simulink model "finishi"  (R2016b)
settings: Solver=ode3  StartTime=0.0  StopTime=850.5  FixedStep=0.01  MaxStep=0.01  RelTol=1e-3  EnableMultiTasking=on
PreLoadFcn:
  | m=5;
  | g=9.8;
  | Jxx=0.1539;
  | Jyy=0.1539;
  | Jzz=0.2634;
  | d=0.4;
  | CT=2.757*10^(-5);
  | CM=4.308*10^(-7);
  | CR=727.36;
  | Wb=173.03;
  | Jm=8.61*10^(-5);
  | Tm=0.0435;
  | Cd=0.712
libraries: simulink x10
settings Model: Creator=StarFly  LastModifiedBy=user
settings DataIOCC: LimitDataPoints=on  SaveFormat=Array
settings OptimizationCC: LifeSpan=inf
settings DebuggingCC: SolverPrmCheckMsg=warning  SFUnexpectedBacktrackingDiag=warning  SFNoUnconditionalDefaultTransitionDiag=warning  SFExecutionAtInitializationDiag=none
settings HardwareCC: ProdBitPerPointer=32  ProdBitPerSizeT=32  ProdBitPerPtrDiffT=32  ProdLargestAtomicFloat=None  ProdIntDivRoundTo=Undefined  ProdEndianess=Unspecified  ProdWordSize=32  ProdHWDeviceType=32-bit Generic
settings ModelReferenceCC: PropagateSignalLabelsOutOfModel=off
settings GRTTargetCC: TargetLangStandard=C89/C90 (ANSI)  GeneratePreprocessorConditionals=Disable all
settings ConfigComp: CovMetricSettings=dw  CovHtmlReporting=on  CovSaveCumulativeToWorkspaceVar=on  CovSaveSingleToWorkspaceVar=on  CovExternalEMLEnable=off  CovSFcnEnable=off

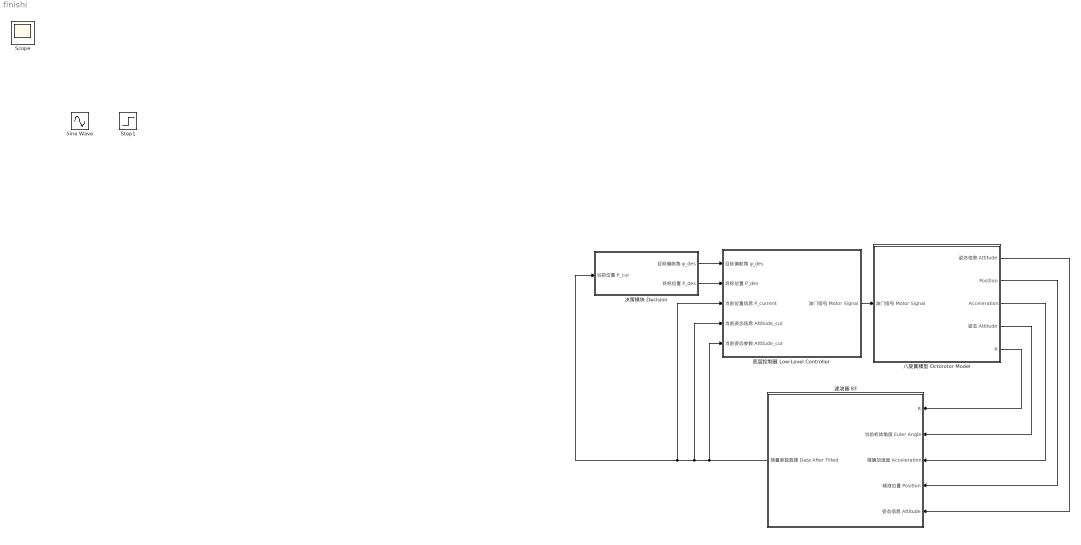
== system finishi ==
  八旋翼模型 Octorotor Model : Subsystem
  决策模块 Decision : Subsystem
  底层控制器 Low-Level Controller : Subsystem
  滤波器 KF : Subsystem
  Scope : Scope
  Sine Wave : Sin  IOType=siggen  SampleTime=0
  Step1 : Step  IOType=siggen  SampleTime=0
  wires:
  滤波器 KF/1(测量参数数据 Data After Filted) -> 底层控制器 Low-Level Controller/4(当前姿态信息 Attitude_cur), 决策模块 Decision/1(当前位置 P_cur), 底层控制器 Low-Level Controller/3(当前位置信息 P_current), 底层控制器 Low-Level Controller/5(当前姿态参数 Attitude_cur)
  八旋翼模型 Octorotor Model/5(R) -> 滤波器 KF/1(R)
  八旋翼模型 Octorotor Model/4(姿态 Attitude) -> 滤波器 KF/2(当前机体角度 Euler Angle)
  八旋翼模型 Octorotor Model/3(Acceleration) -> 滤波器 KF/3(精确加速度 Acceleration)
  八旋翼模型 Octorotor Model/2(Position) -> 滤波器 KF/4(精准位置 Position)
  八旋翼模型 Octorotor Model/1(姿态信息 Attitude) -> 滤波器 KF/5(姿态信息 Attitude)
  决策模块 Decision/1(目标偏航角 ψ_des) -> 底层控制器 Low-Level Controller/1(目标偏航角 ψ_des)
  决策模块 Decision/2(目标位置 P_des) -> 底层控制器 Low-Level Controller/2(目标位置 P_des)
  底层控制器 Low-Level Controller/1(油门信号 Motor Signal) -> 八旋翼模型 Octorotor Model/1(油门信号 Motor Signal)

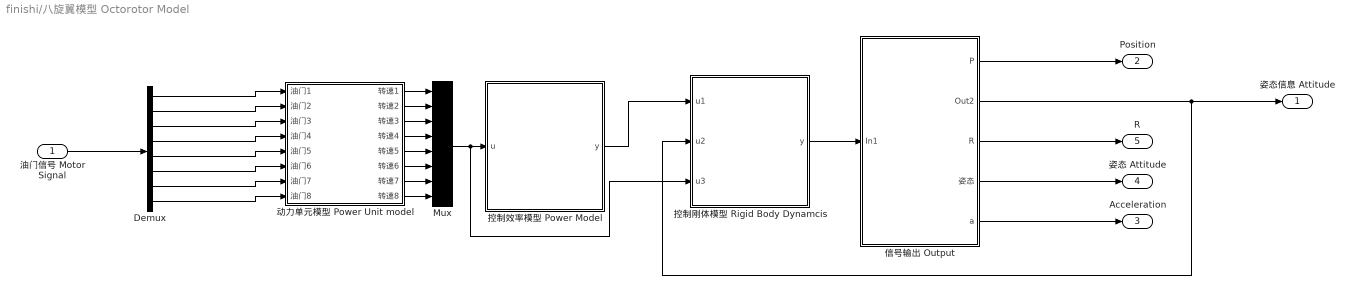
== system finishi/八旋翼模型 Octorotor Model ==
  油门信号 Motor Signal : Inport
  Demux : Demux  Outputs=8
  Mux : Mux  Inputs=8
  信号输出 Output : Subsystem
  动力单元模型 Power Unit model : Subsystem
  控制刚体模型 Rigid Body Dynamcis : MATLAB Function  TreatAsAtomicUnit=on
  控制效率模型 Power Model : MATLAB Function  TreatAsAtomicUnit=on
  姿态信息 Attitude : Outport
  Position : Outport  Port=2
  Acceleration : Outport  Port=3
  姿态 Attitude : Outport  Port=4
  R : Outport  Port=5
  wires:
  动力单元模型 Power Unit model/6(转速6) -> Mux/6
  动力单元模型 Power Unit model/7(转速7) -> Mux/7
  动力单元模型 Power Unit model/8(转速8) -> Mux/8
  动力单元模型 Power Unit model/3(转速3) -> Mux/3
  动力单元模型 Power Unit model/2(转速2) -> Mux/2
  Demux/5 -> 动力单元模型 Power Unit model/5(油门5)
  Mux/1 -> 控制效率模型 Power Model/1(u), 控制刚体模型 Rigid Body Dynamcis/3(u3)
  Demux/3 -> 动力单元模型 Power Unit model/3(油门3)
  Demux/1 -> 动力单元模型 Power Unit model/1(油门1)
  Demux/2 -> 动力单元模型 Power Unit model/2(油门2)
  Demux/6 -> 动力单元模型 Power Unit model/6(油门6)
  动力单元模型 Power Unit model/4(转速4) -> Mux/4
  动力单元模型 Power Unit model/1(转速1) -> Mux/1
  控制效率模型 Power Model/1(y) -> 控制刚体模型 Rigid Body Dynamcis/1(u1)
  Demux/7 -> 动力单元模型 Power Unit model/7(油门7)
  Demux/8 -> 动力单元模型 Power Unit model/8(油门8)
  油门信号 Motor Signal/1 -> Demux/1
  Demux/4 -> 动力单元模型 Power Unit model/4(油门4)
  动力单元模型 Power Unit model/5(转速5) -> Mux/5
  信号输出 Output/2(Out2) -> 控制刚体模型 Rigid Body Dynamcis/2(u2), 姿态信息 Attitude/1
  控制刚体模型 Rigid Body Dynamcis/1(y) -> 信号输出 Output/1(In1)
  信号输出 Output/1(P) -> Position/1
  信号输出 Output/3(R) -> R/1
  信号输出 Output/4(姿态) -> 姿态 Attitude/1
  信号输出 Output/5(a) -> Acceleration/1

== system finishi/决策模块 Decision ==
  当前位置 P_cur : Inport
  Clock : Clock
  决策 Decision : MATLAB Function  TreatAsAtomicUnit=on
  目标psi : Constant  Value=0
  目标偏航角 ψ_des : Outport
  目标位置 P_des : Outport  Port=2
  wires:
  当前位置 P_cur/1 -> 决策 Decision/1(u1)
  Clock/1 -> 决策 Decision/2(u2)
  决策 Decision/1(y) -> 目标位置 P_des/1
  目标psi/1 -> 目标偏航角 ψ_des/1

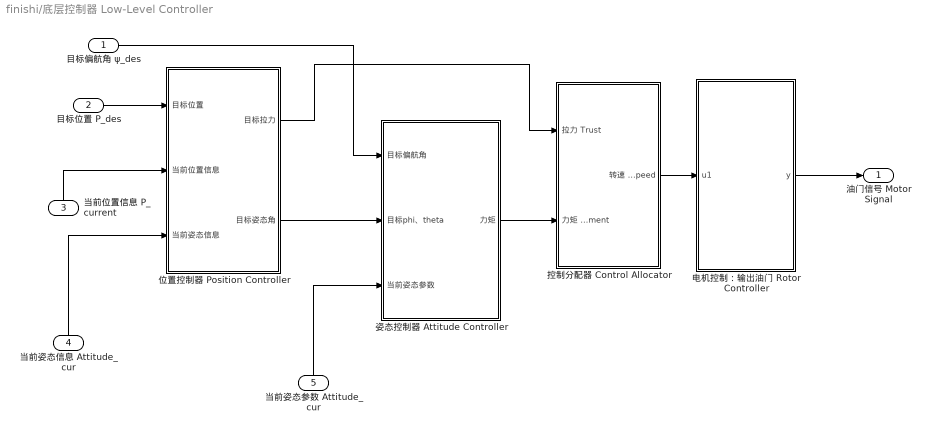
== system finishi/底层控制器 Low-Level Controller ==
  目标偏航角 ψ_des : Inport
  目标位置 P_des : Inport  Port=2
  当前位置信息 P_current : Inport  Port=3
  当前姿态信息 Attitude_cur : Inport  Port=4
  当前姿态参数 Attitude_cur : Inport  Port=5
  位置控制器 Position Controller : Subsystem
  姿态控制器 Attitude Controller : Subsystem
  "控制分配器 Control Allocator " : Subsystem
  电机控制：输出油门 Rotor Controller : MATLAB Function  TreatAsAtomicUnit=on
  油门信号 Motor Signal : Outport
  wires:
  目标偏航角 ψ_des/1 -> 姿态控制器 Attitude Controller/1(目标偏航角)
  目标位置 P_des/1 -> 位置控制器 Position Controller/1(目标位置)
  当前姿态参数 Attitude_cur/1 -> 姿态控制器 Attitude Controller/3(当前姿态参数)
  当前姿态信息 Attitude_cur/1 -> 位置控制器 Position Controller/3(当前姿态信息)
  位置控制器 Position Controller/1(目标拉力) -> "控制分配器 Control Allocator "/1(拉力 Trust)
  位置控制器 Position Controller/2(目标姿态角) -> 姿态控制器 Attitude Controller/2(目标phi、theta)
  当前位置信息 P_current/1 -> 位置控制器 Position Controller/2(当前位置信息)
  姿态控制器 Attitude Controller/1(力矩) -> "控制分配器 Control Allocator "/2("力矩 Moment ")
  电机控制：输出油门 Rotor Controller/1(y) -> 油门信号 Motor Signal/1
  "控制分配器 Control Allocator "/1("转速 Motor speed ") -> 电机控制：输出油门 Rotor Controller/1(u1)

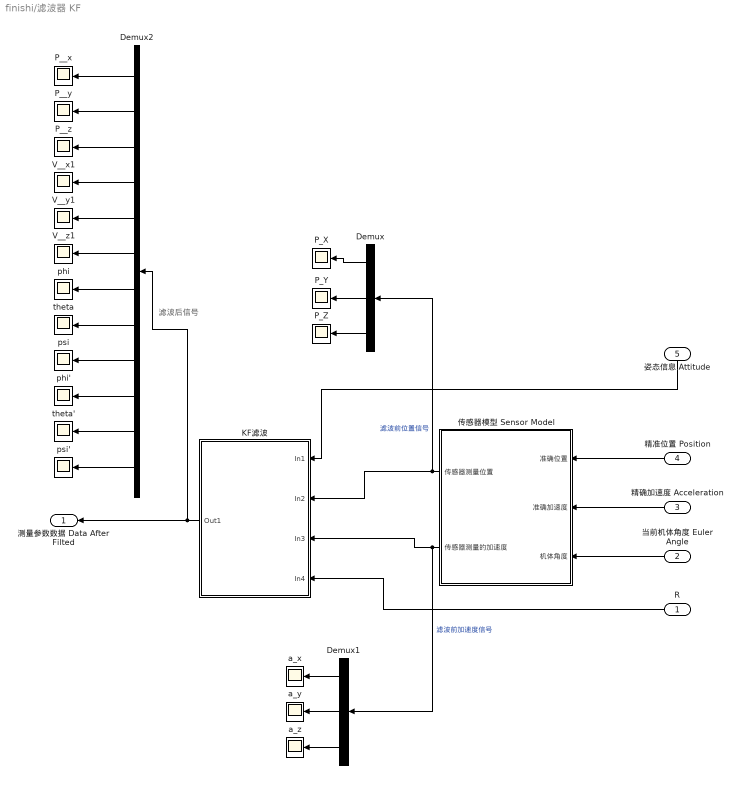
== system finishi/滤波器 KF ==
  note: 滤波后信号
  R : Inport
  当前机体角度 Euler Angle : Inport  Port=2
  精确加速度 Acceleration : Inport  Port=3
  精准位置 Position : Inport  Port=4
  姿态信息 Attitude : Inport  Port=5
  Demux : Demux  Outputs=3
  Demux1 : Demux  Outputs=3
  Demux2 : Demux  Outputs=12
  KF滤波 : Subsystem
  P_X : Scope
  P_Y : Scope
  P_Z : Scope
  P__x : Scope
  P__y : Scope
  P__z : Scope
  V__x1 : Scope
  V__y1 : Scope
  V__z1 : Scope
  a_x : Scope
  a_y : Scope
  a_z : Scope
  phi : Scope
  phi' : Scope
  psi : Scope
  psi' : Scope
  theta : Scope
  theta' : Scope
  传感器模型 Sensor Model : Subsystem
  测量参数数据 Data After Filted : Outport
  wires:
  精准位置 Position/1 -> 传感器模型 Sensor Model/1(准确位置)
  精确加速度 Acceleration/1 -> 传感器模型 Sensor Model/2(准确加速度)
  当前机体角度 Euler Angle/1 -> 传感器模型 Sensor Model/3(机体角度)
  姿态信息 Attitude/1 -> KF滤波/1(In1)
  传感器模型 Sensor Model/1(传感器测量位置) -> Demux/1, KF滤波/2(In2)  "滤波前位置信号"
  R/1 -> KF滤波/4(In4)
  KF滤波/1(Out1) -> Demux2/1, 测量参数数据 Data After Filted/1
  Demux/1 -> P_X/1
  Demux/2 -> P_Y/1
  Demux/3 -> P_Z/1
  传感器模型 Sensor Model/2(传感器测量的加速度) -> Demux1/1, KF滤波/3(In3)  "滤波前加速度信号"
  Demux1/1 -> a_x/1
  Demux1/2 -> a_y/1
  Demux1/3 -> a_z/1
  Demux2/1 -> P__x/1
  Demux2/2 -> P__y/1
  Demux2/3 -> P__z/1
  Demux2/4 -> V__x1/1
  Demux2/5 -> V__y1/1
  Demux2/6 -> V__z1/1
  Demux2/7 -> phi/1
  Demux2/8 -> theta/1
  Demux2/9 -> psi/1
  Demux2/10 -> phi'/1
  Demux2/11 -> theta'/1
  Demux2/12 -> psi'/1

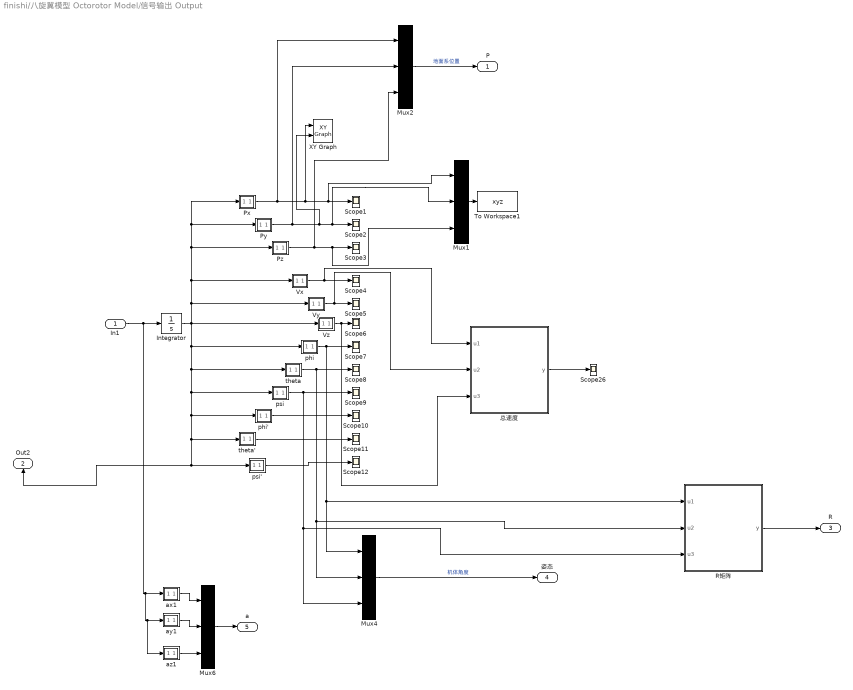
== system finishi/八旋翼模型 Octorotor Model/信号输出 Output ==
  In1 : Inport
  Integrator : Integrator  InitialCondition=[0;0;0;0;0;0;0;0;0;0;0;0]
  Mux{1..2,4,6} (4 alike) : Mux  Inputs=3
  Px : MATLAB Function  TreatAsAtomicUnit=on
  Py : MATLAB Function  TreatAsAtomicUnit=on
  Pz : MATLAB Function  TreatAsAtomicUnit=on
  R矩阵 : MATLAB Function  TreatAsAtomicUnit=on
  Scope{1..12,26} (13 alike) : Scope
  To Workspace1 : ToWorkspace  VariableName=xyz  SampleTime=-1
  Vx : MATLAB Function  TreatAsAtomicUnit=on
  Vy : MATLAB Function  TreatAsAtomicUnit=on
  Vz : MATLAB Function  TreatAsAtomicUnit=on
  XY Graph : simulink/Sinks/XY Graph  xmin=-1  xmax=50  ymin=-1  ymax=120  st=-1
  ax1 : MATLAB Function  TreatAsAtomicUnit=on
  ay1 : MATLAB Function  TreatAsAtomicUnit=on
  az1 : MATLAB Function  TreatAsAtomicUnit=on
  phi : MATLAB Function  TreatAsAtomicUnit=on
  phi' : MATLAB Function  TreatAsAtomicUnit=on
  psi : MATLAB Function  TreatAsAtomicUnit=on
  psi' : MATLAB Function  TreatAsAtomicUnit=on
  theta : MATLAB Function  TreatAsAtomicUnit=on
  theta' : MATLAB Function  TreatAsAtomicUnit=on
  "总速度 " : MATLAB Function  TreatAsAtomicUnit=on
  P : Outport
  Out2 : Outport  Port=2
  R : Outport  Port=3
  姿态 : Outport  Port=4
  a : Outport  Port=5
  wires:
  Vx/1(y) -> "总速度 "/1(u1), Scope4/1
  theta'/1(y) -> Scope11/1
  In1/1 -> az1/1(u), ay1/1(u), ax1/1(u), Integrator/1
  Py/1(y) -> Mux2/2, XY Graph/2, Mux1/2, Scope2/1
  Vy/1(y) -> Scope5/1, "总速度 "/2(u2)
  phi'/1(y) -> Scope10/1
  Vz/1(y) -> "总速度 "/3(u3), Scope6/1
  phi/1(y) -> R矩阵/1(u1), Mux4/1, Scope7/1
  psi/1(y) -> R矩阵/3(u3), Mux4/3, Scope9/1
  Pz/1(y) -> Mux2/3, Mux1/3, Scope3/1
  theta/1(y) -> R矩阵/2(u2), Mux4/2, Scope8/1
  Px/1(y) -> Mux2/1, XY Graph/1, Mux1/1, Scope1/1
  psi'/1(y) -> Scope12/1
  "总速度 "/1(y) -> Scope26/1
  Integrator/1 -> Out2/1, psi'/1(u), theta'/1(u), phi'/1(u), psi/1(u), theta/1(u), phi/1(u), Vz/1(u), Vx/1(u), Px/1(u), Py/1(u), Pz/1(u), Vy/1(u)
  Mux2/1 -> P/1  "地面系位置"
  Mux6/1 -> a/1
  R矩阵/1(y) -> R/1
  Mux4/1 -> 姿态/1  "机体角度"
  ay1/1(y) -> Mux6/2
  az1/1(y) -> Mux6/3
  Mux1/1 -> To Workspace1/1
  ax1/1(y) -> Mux6/1

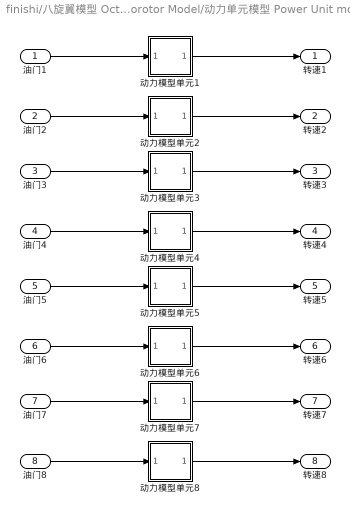
== system finishi/八旋翼模型 Octorotor Model/动力单元模型 Power Unit model ==
  油门1 : Inport
  油门2 : Inport  Port=2
  油门3 : Inport  Port=3
  油门4 : Inport  Port=4
  油门5 : Inport  Port=5
  油门6 : Inport  Port=6
  油门7 : Inport  Port=7
  油门8 : Inport  Port=8
  动力模型单元1 : Subsystem
  动力模型单元2 : Subsystem
  动力模型单元3 : Subsystem
  动力模型单元4 : Subsystem
  动力模型单元5 : Subsystem
  动力模型单元6 : Subsystem
  动力模型单元7 : Subsystem
  动力模型单元8 : Subsystem
  转速1 : Outport
  转速2 : Outport  Port=2
  转速3 : Outport  Port=3
  转速4 : Outport  Port=4
  转速5 : Outport  Port=5
  转速6 : Outport  Port=6
  转速7 : Outport  Port=7
  转速8 : Outport  Port=8
  wires:
  油门1/1 -> 动力模型单元1/1(In1)
  动力模型单元1/1(Out1) -> 转速1/1
  油门2/1 -> 动力模型单元2/1(In1)
  动力模型单元2/1(Out1) -> 转速2/1
  油门3/1 -> 动力模型单元3/1(In1)
  动力模型单元3/1(Out1) -> 转速3/1
  油门4/1 -> 动力模型单元4/1(In1)
  动力模型单元4/1(Out1) -> 转速4/1
  油门5/1 -> 动力模型单元5/1(In1)
  动力模型单元5/1(Out1) -> 转速5/1
  油门6/1 -> 动力模型单元6/1(In1)
  动力模型单元6/1(Out1) -> 转速6/1
  油门7/1 -> 动力模型单元7/1(In1)
  动力模型单元7/1(Out1) -> 转速7/1
  油门8/1 -> 动力模型单元8/1(In1)
  动力模型单元8/1(Out1) -> 转速8/1

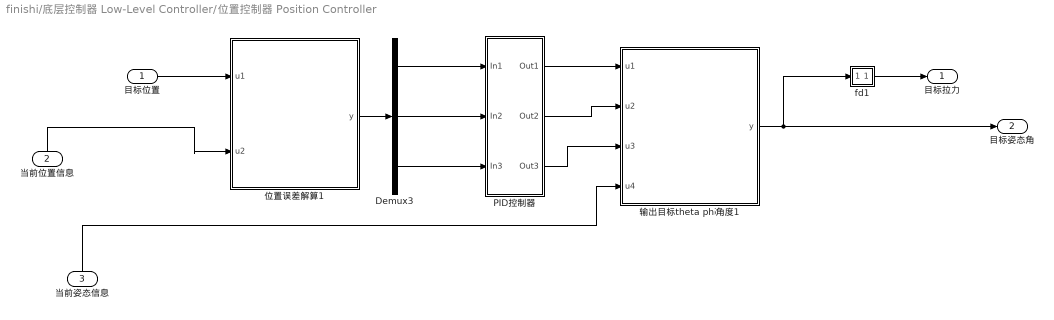
== system finishi/底层控制器 Low-Level Controller/位置控制器 Position Controller ==
  目标位置 : Inport
  当前位置信息 : Inport  Port=2
  当前姿态信息 : Inport  Port=3
  Demux3 : Demux  Outputs=3
  PID控制器 : Subsystem
  fd1 : MATLAB Function  TreatAsAtomicUnit=on
  位置误差解算1 : MATLAB Function  TreatAsAtomicUnit=on
  输出目标theta phi角度1 : MATLAB Function  TreatAsAtomicUnit=on
  目标拉力 : Outport
  目标姿态角 : Outport  Port=2
  wires:
  目标位置/1 -> 位置误差解算1/1(u1)
  fd1/1(y) -> 目标拉力/1
  位置误差解算1/1(y) -> Demux3/1
  输出目标theta phi角度1/1(y) -> fd1/1(u), 目标姿态角/1
  当前位置信息/1 -> 位置误差解算1/2(u2)
  当前姿态信息/1 -> 输出目标theta phi角度1/4(u4)
  Demux3/1 -> PID控制器/1(In1)
  Demux3/2 -> PID控制器/2(In2)
  Demux3/3 -> PID控制器/3(In3)
  PID控制器/1(Out1) -> 输出目标theta phi角度1/1(u1)
  PID控制器/2(Out2) -> 输出目标theta phi角度1/2(u2)
  PID控制器/3(Out3) -> 输出目标theta phi角度1/3(u3)

== system finishi/底层控制器 Low-Level Controller/姿态控制器 Attitude Controller ==
  目标偏航角 : Inport
  目标phi、theta : Inport  Port=2
  当前姿态参数 : Inport  Port=3
  PID控制器 : Subsystem
  姿态误差解算1 : MATLAB Function  TreatAsAtomicUnit=on
  输出目标力矩1 : MATLAB Function  TreatAsAtomicUnit=on
  力矩 : Outport
  wires:
  目标偏航角/1 -> 姿态误差解算1/2(u2)
  当前姿态参数/1 -> 姿态误差解算1/3(u3)
  目标phi、theta/1 -> 姿态误差解算1/1(u1)
  输出目标力矩1/1(y) -> 力矩/1
  姿态误差解算1/1(y) -> PID控制器/1(In1)
  PID控制器/1(Out1) -> 输出目标力矩1/1(u1)
  PID控制器/2(Out2) -> 输出目标力矩1/2(u2)
  PID控制器/3(Out3) -> 输出目标力矩1/3(u3)

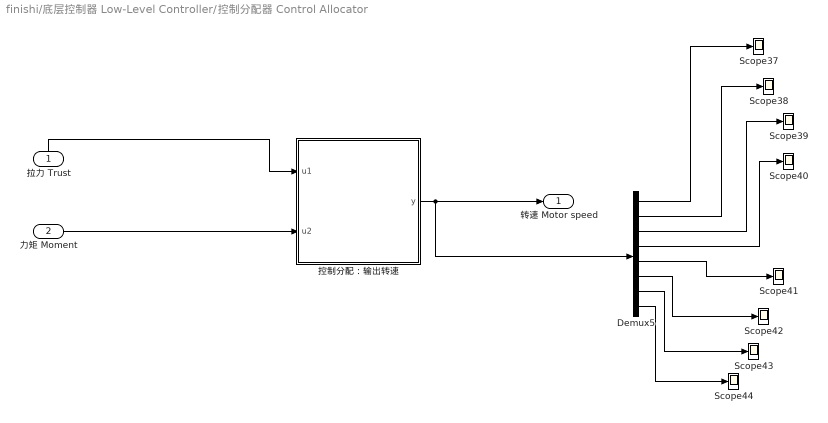
== system finishi/底层控制器 Low-Level Controller/控制分配器 Control Allocator  ==
  拉力 Trust : Inport
  "力矩 Moment " : Inport  Port=2
  Demux5 : Demux  Outputs=8
  Scope{37..44} (8 alike) : Scope
  控制分配：输出转速 : MATLAB Function  TreatAsAtomicUnit=on
  "转速 Motor speed " : Outport
  wires:
  控制分配：输出转速/1(y) -> "转速 Motor speed "/1, Demux5/1
  "力矩 Moment "/1 -> 控制分配：输出转速/2(u2)
  Demux5/1 -> Scope37/1
  Demux5/3 -> Scope39/1
  Demux5/5 -> Scope41/1
  Demux5/8 -> Scope44/1
  Demux5/2 -> Scope38/1
  Demux5/4 -> Scope40/1
  Demux5/7 -> Scope43/1
  Demux5/6 -> Scope42/1
  拉力 Trust/1 -> 控制分配：输出转速/1(u1)

== system finishi/滤波器 KF/KF滤波 ==
  In1 : Inport
  In2 : Inport  Port=2
  In3 : Inport  Port=3
  In4 : Inport  Port=4
  KF : Subsystem
  位置、速度、姿态信息整合 : Subsystem
  Out1 : Outport
  wires:
  KF/1(滤波后位置) -> 位置、速度、姿态信息整合/2(In2)
  In4/1 -> KF/3(R矩阵)
  In3/1 -> KF/2(传感器加速度)
  In2/1 -> KF/1(传感器位置)
  位置、速度、姿态信息整合/1(Out1) -> Out1/1
  KF/2(滤波后速度) -> 位置、速度、姿态信息整合/3(In3)
  In1/1 -> 位置、速度、姿态信息整合/1(In1)

== system finishi/滤波器 KF/传感器模型 Sensor Model ==
  准确位置 : Inport
  准确加速度 : Inport  Port=2
  机体角度 : Inport  Port=3
  GPS模型 : Subsystem
  加速度计模型 : Subsystem
  传感器测量位置 : Outport
  传感器测量的加速度 : Outport  Port=2
  wires:
  准确加速度/1 -> 加速度计模型/1(准确加速度)
  机体角度/1 -> 加速度计模型/2(机体角度)
  加速度计模型/1(传感器测量的加速度) -> 传感器测量的加速度/1
  准确位置/1 -> GPS模型/1(In1)
  GPS模型/1(Out1) -> 传感器测量位置/1

== system finishi/八旋翼模型 Octorotor Model/动力单元模型 Power Unit model/动力模型单元1 ==
  In1 : Inport
  CR : Constant  Value=CR
  Product : Product
  Wb : Constant  Value=Wb
  Wss : Sum
  动态响应 : TransferFcn  Denominator=[Tm 1]
  Out1 : Outport
  wires:
  In1/1 -> Product/2
  Wss/1 -> 动态响应/1
  动态响应/1 -> Out1/1
  Wb/1 -> Wss/1
  CR/1 -> Product/1
  Product/1 -> Wss/2

== system finishi/八旋翼模型 Octorotor Model/动力单元模型 Power Unit model/动力模型单元2 ==
  In1 : Inport
  CR : Constant  Value=CR
  Product : Product
  Wb : Constant  Value=Wb
  Wss : Sum
  动态响应 : TransferFcn  Denominator=[Tm 1]
  Out1 : Outport
  wires:
  Product/1 -> Wss/2
  CR/1 -> Product/1
  Wb/1 -> Wss/1
  动态响应/1 -> Out1/1
  Wss/1 -> 动态响应/1
  In1/1 -> Product/2

== system finishi/八旋翼模型 Octorotor Model/动力单元模型 Power Unit model/动力模型单元3 ==
  In1 : Inport
  CR : Constant  Value=CR
  Product : Product
  Wb : Constant  Value=Wb
  Wss : Sum
  动态响应 : TransferFcn  Denominator=[Tm 1]
  Out1 : Outport
  wires:
  In1/1 -> Product/2
  Wss/1 -> 动态响应/1
  动态响应/1 -> Out1/1
  Wb/1 -> Wss/1
  CR/1 -> Product/1
  Product/1 -> Wss/2

== system finishi/八旋翼模型 Octorotor Model/动力单元模型 Power Unit model/动力模型单元4 ==
  In1 : Inport
  CR : Constant  Value=CR
  Product : Product
  Wb : Constant  Value=Wb
  Wss : Sum
  动态响应 : TransferFcn  Denominator=[Tm 1]
  Out1 : Outport
  wires:
  Product/1 -> Wss/2
  CR/1 -> Product/1
  Wb/1 -> Wss/1
  动态响应/1 -> Out1/1
  Wss/1 -> 动态响应/1
  In1/1 -> Product/2

== system finishi/八旋翼模型 Octorotor Model/动力单元模型 Power Unit model/动力模型单元5 ==
  In1 : Inport
  CR : Constant  Value=CR
  Product : Product
  Wb : Constant  Value=Wb
  Wss : Sum
  动态响应 : TransferFcn  Denominator=[Tm 1]
  Out1 : Outport
  wires:
  In1/1 -> Product/2
  Wss/1 -> 动态响应/1
  动态响应/1 -> Out1/1
  Wb/1 -> Wss/1
  CR/1 -> Product/1
  Product/1 -> Wss/2

== system finishi/八旋翼模型 Octorotor Model/动力单元模型 Power Unit model/动力模型单元6 ==
  In1 : Inport
  CR : Constant  Value=CR
  Product : Product
  Wb : Constant  Value=Wb
  Wss : Sum
  动态响应 : TransferFcn  Denominator=[Tm 1]
  Out1 : Outport
  wires:
  Product/1 -> Wss/2
  CR/1 -> Product/1
  Wb/1 -> Wss/1
  动态响应/1 -> Out1/1
  Wss/1 -> 动态响应/1
  In1/1 -> Product/2

== system finishi/八旋翼模型 Octorotor Model/动力单元模型 Power Unit model/动力模型单元7 ==
  In1 : Inport
  CR : Constant  Value=CR
  Product : Product
  Wb : Constant  Value=Wb
  Wss : Sum
  动态响应 : TransferFcn  Denominator=[Tm 1]
  Out1 : Outport
  wires:
  In1/1 -> Product/2
  Wss/1 -> 动态响应/1
  动态响应/1 -> Out1/1
  Wb/1 -> Wss/1
  CR/1 -> Product/1
  Product/1 -> Wss/2

== system finishi/八旋翼模型 Octorotor Model/动力单元模型 Power Unit model/动力模型单元8 ==
  In1 : Inport
  CR : Constant  Value=CR
  Product : Product
  Wb : Constant  Value=Wb
  Wss : Sum
  动态响应 : TransferFcn  Denominator=[Tm 1]
  Out1 : Outport
  wires:
  Product/1 -> Wss/2
  CR/1 -> Product/1
  Wb/1 -> Wss/1
  动态响应/1 -> Out1/1
  Wss/1 -> 动态响应/1
  In1/1 -> Product/2

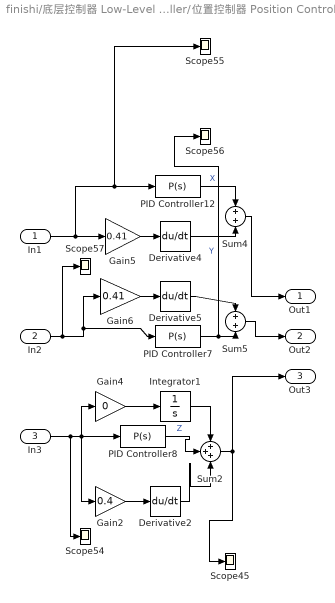
== system finishi/底层控制器 Low-Level Controller/位置控制器 Position Controller/PID控制器 ==
  In1 : Inport
  In2 : Inport  Port=2
  In3 : Inport  Port=3
  Derivative2 : Derivative
  Derivative4 : Derivative  CoefficientInTFapproximation=4.8
  Derivative5 : Derivative
  Gain2 : Gain  Gain=0.4
  Gain4 : Gain  Gain=0
  Gain5 : Gain  Gain=0.41
  Gain6 : Gain  Gain=0.41
  Integrator1 : Integrator
  PID Controller12 : simulink/Continuous/PID Controller  Controller=P  TimeDomain=Continuous-time  SampleTime=-1  IntegratorMethod=Forward Euler  FilterMethod=Forward Euler  Form=Parallel  UseFilter=on  ControllerParametersSource=internal  P=8  I=0  D=1  N=100  InitialConditionSource=internal  InitialConditionForIntegrator=0  InitialConditionForFilter=0  ExternalReset=none  LimitOutput=off  UpperSaturationLimit=inf  LowerSaturationLimit=-inf  LinearizeAsGain=on  AntiWindupMode=none  Kb=1  TrackingMode=off  Kt=1  PParamMin=[]  PParamMax=[]  IParamMin=[]  IParamMax=[]  DParamMin=[]  DParamMax=[]  NParamMin=[]  NParamMax=[]  KbParamMin=[]  KbParamMax=[]  KtParamMin=[]  KtParamMax=[]  POutMin=[]  POutMax=[]  IOutMin=[]  IOutMax=[]  DOutMin=[]  DOutMax=[]  NOutMin=[]  NOutMax=[]  KbOutMin=[]  KbOutMax=[]  KtOutMin=[]  KtOutMax=[]  IntegratorOutMin=[]  IntegratorOutMax=[]  FilterOutMin=[]  FilterOutMax=[]  SumOutMin=[]  SumOutMax=[]  SumI1OutMin=[]  SumI1OutMax=[]  SumI2OutMin=[]  SumI2OutMax=[]  SumI3OutMin=[]  SumI3OutMax=[]  SumDOutMin=[]  SumDOutMax=[]  SaturationOutMin=[]  SaturationOutMax=[]  IntegratorContinuousStateAttributes=''  IntegratorStateMustResolveToSignalObject=off  IntegratorRTWStateStorageClass=Auto  FilterContinuousStateAttributes=''  FilterStateMustResolveToSignalObject=off  FilterRTWStateStorageClass=Auto  DifferentiatorICPrevScaledInput=0  DifferentiatorOutMin=[]  DifferentiatorOutMax=[]
  PID Controller7 : simulink/Continuous/PID Controller  Controller=P  TimeDomain=Continuous-time  SampleTime=-1  IntegratorMethod=Forward Euler  FilterMethod=Forward Euler  Form=Parallel  UseFilter=on  ControllerParametersSource=internal  P=8  I=0  D=1  N=100  InitialConditionSource=internal  InitialConditionForIntegrator=0  InitialConditionForFilter=0  ExternalReset=none  LimitOutput=off  UpperSaturationLimit=inf  LowerSaturationLimit=-inf  LinearizeAsGain=on  AntiWindupMode=none  Kb=1  TrackingMode=off  Kt=1  PParamMin=[]  PParamMax=[]  IParamMin=[]  IParamMax=[]  DParamMin=[]  DParamMax=[]  NParamMin=[]  NParamMax=[]  KbParamMin=[]  KbParamMax=[]  KtParamMin=[]  KtParamMax=[]  POutMin=[]  POutMax=[]  IOutMin=[]  IOutMax=[]  DOutMin=[]  DOutMax=[]  NOutMin=[]  NOutMax=[]  KbOutMin=[]  KbOutMax=[]  KtOutMin=[]  KtOutMax=[]  IntegratorOutMin=[]  IntegratorOutMax=[]  FilterOutMin=[]  FilterOutMax=[]  SumOutMin=[]  SumOutMax=[]  SumI1OutMin=[]  SumI1OutMax=[]  SumI2OutMin=[]  SumI2OutMax=[]  SumI3OutMin=[]  SumI3OutMax=[]  SumDOutMin=[]  SumDOutMax=[]  SaturationOutMin=[]  SaturationOutMax=[]  IntegratorContinuousStateAttributes=''  IntegratorStateMustResolveToSignalObject=off  IntegratorRTWStateStorageClass=Auto  FilterContinuousStateAttributes=''  FilterStateMustResolveToSignalObject=off  FilterRTWStateStorageClass=Auto  DifferentiatorICPrevScaledInput=0  DifferentiatorOutMin=[]  DifferentiatorOutMax=[]
  PID Controller8 : simulink/Continuous/PID Controller  Controller=P  TimeDomain=Continuous-time  SampleTime=-1  IntegratorMethod=Forward Euler  FilterMethod=Forward Euler  Form=Parallel  UseFilter=on  ControllerParametersSource=internal  P=20  I=0  D=1  N=100  InitialConditionSource=internal  InitialConditionForIntegrator=0  InitialConditionForFilter=0  ExternalReset=none  LimitOutput=off  UpperSaturationLimit=inf  LowerSaturationLimit=-inf  LinearizeAsGain=on  AntiWindupMode=none  Kb=1  TrackingMode=off  Kt=1  PParamMin=[]  PParamMax=[]  IParamMin=[]  IParamMax=[]  DParamMin=[]  DParamMax=[]  NParamMin=[]  NParamMax=[]  KbParamMin=[]  KbParamMax=[]  KtParamMin=[]  KtParamMax=[]  POutMin=[]  POutMax=[]  IOutMin=[]  IOutMax=[]  DOutMin=[]  DOutMax=[]  NOutMin=[]  NOutMax=[]  KbOutMin=[]  KbOutMax=[]  KtOutMin=[]  KtOutMax=[]  IntegratorOutMin=[]  IntegratorOutMax=[]  FilterOutMin=[]  FilterOutMax=[]  SumOutMin=[]  SumOutMax=[]  SumI1OutMin=[]  SumI1OutMax=[]  SumI2OutMin=[]  SumI2OutMax=[]  SumI3OutMin=[]  SumI3OutMax=[]  SumDOutMin=[]  SumDOutMax=[]  SaturationOutMin=[]  SaturationOutMax=[]  IntegratorContinuousStateAttributes=''  IntegratorStateMustResolveToSignalObject=off  IntegratorRTWStateStorageClass=Auto  FilterContinuousStateAttributes=''  FilterStateMustResolveToSignalObject=off  FilterRTWStateStorageClass=Auto  DifferentiatorICPrevScaledInput=0  DifferentiatorOutMin=[]  DifferentiatorOutMax=[]
  Scope{45,54..57} (5 alike) : Scope
  Sum2 : Sum  Inputs=+++
  Sum4 : Sum
  Sum5 : Sum
  Out1 : Outport
  Out2 : Outport  Port=2
  Out3 : Outport  Port=3
  wires:
  PID Controller7/1 -> Sum5/2, Scope56/1  "Y"
  In1/1 -> Gain5/1, Scope55/1, PID Controller12/1
  PID Controller8/1 -> Sum2/2  "Z"
  In3/1 -> Scope54/1, Gain4/1, Gain2/1, PID Controller8/1
  PID Controller12/1 -> Sum4/1  "X"
  In2/1 -> Gain6/1, PID Controller7/1, Scope57/1
  Derivative2/1 -> Sum2/3
  Sum2/1 -> Out3/1, Scope45/1
  Gain2/1 -> Derivative2/1
  Derivative5/1 -> Sum5/1
  Gain5/1 -> Derivative4/1
  Gain4/1 -> Integrator1/1
  Gain6/1 -> Derivative5/1
  Sum5/1 -> Out2/1
  Sum4/1 -> Out1/1
  Integrator1/1 -> Sum2/1
  Derivative4/1 -> Sum4/2

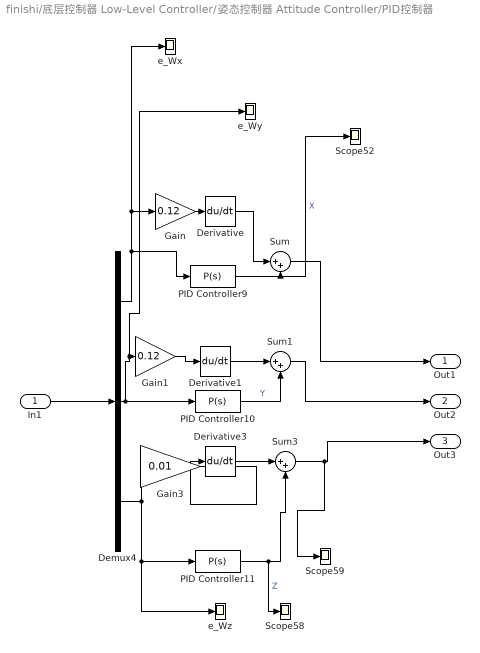
== system finishi/底层控制器 Low-Level Controller/姿态控制器 Attitude Controller/PID控制器 ==
  In1 : Inport
  Demux4 : Demux  Outputs=3
  Derivative : Derivative
  Derivative1 : Derivative
  Derivative3 : Derivative
  Gain : Gain  Gain=0.12
  Gain1 : Gain  Gain=0.12
  Gain3 : Gain  Gain=0.01
  PID Controller10 : simulink/Continuous/PID Controller  Controller=P  TimeDomain=Continuous-time  SampleTime=-1  IntegratorMethod=Forward Euler  FilterMethod=Forward Euler  Form=Parallel  UseFilter=on  ControllerParametersSource=internal  P=8  I=0  D=1  N=100  InitialConditionSource=internal  InitialConditionForIntegrator=0  InitialConditionForFilter=0  ExternalReset=none  LimitOutput=off  UpperSaturationLimit=inf  LowerSaturationLimit=-inf  LinearizeAsGain=on  AntiWindupMode=none  Kb=1  TrackingMode=off  Kt=1  PParamMin=[]  PParamMax=[]  IParamMin=[]  IParamMax=[]  DParamMin=[]  DParamMax=[]  NParamMin=[]  NParamMax=[]  KbParamMin=[]  KbParamMax=[]  KtParamMin=[]  KtParamMax=[]  POutMin=[]  POutMax=[]  IOutMin=[]  IOutMax=[]  DOutMin=[]  DOutMax=[]  NOutMin=[]  NOutMax=[]  KbOutMin=[]  KbOutMax=[]  KtOutMin=[]  KtOutMax=[]  IntegratorOutMin=[]  IntegratorOutMax=[]  FilterOutMin=[]  FilterOutMax=[]  SumOutMin=[]  SumOutMax=[]  SumI1OutMin=[]  SumI1OutMax=[]  SumI2OutMin=[]  SumI2OutMax=[]  SumI3OutMin=[]  SumI3OutMax=[]  SumDOutMin=[]  SumDOutMax=[]  SaturationOutMin=[]  SaturationOutMax=[]  IntegratorContinuousStateAttributes=''  IntegratorStateMustResolveToSignalObject=off  IntegratorRTWStateStorageClass=Auto  FilterContinuousStateAttributes=''  FilterStateMustResolveToSignalObject=off  FilterRTWStateStorageClass=Auto  DifferentiatorICPrevScaledInput=0  DifferentiatorOutMin=[]  DifferentiatorOutMax=[]
  PID Controller11 : simulink/Continuous/PID Controller  Controller=P  TimeDomain=Continuous-time  SampleTime=-1  IntegratorMethod=Forward Euler  FilterMethod=Forward Euler  Form=Parallel  UseFilter=on  ControllerParametersSource=internal  P=2.4475  I=0  D=1  N=100  InitialConditionSource=internal  InitialConditionForIntegrator=0  InitialConditionForFilter=0  ExternalReset=none  LimitOutput=off  UpperSaturationLimit=inf  LowerSaturationLimit=-inf  LinearizeAsGain=on  AntiWindupMode=none  Kb=1  TrackingMode=off  Kt=1  PParamMin=[]  PParamMax=[]  IParamMin=[]  IParamMax=[]  DParamMin=[]  DParamMax=[]  NParamMin=[]  NParamMax=[]  KbParamMin=[]  KbParamMax=[]  KtParamMin=[]  KtParamMax=[]  POutMin=[]  POutMax=[]  IOutMin=[]  IOutMax=[]  DOutMin=[]  DOutMax=[]  NOutMin=[]  NOutMax=[]  KbOutMin=[]  KbOutMax=[]  KtOutMin=[]  KtOutMax=[]  IntegratorOutMin=[]  IntegratorOutMax=[]  FilterOutMin=[]  FilterOutMax=[]  SumOutMin=[]  SumOutMax=[]  SumI1OutMin=[]  SumI1OutMax=[]  SumI2OutMin=[]  SumI2OutMax=[]  SumI3OutMin=[]  SumI3OutMax=[]  SumDOutMin=[]  SumDOutMax=[]  SaturationOutMin=[]  SaturationOutMax=[]  IntegratorContinuousStateAttributes=''  IntegratorStateMustResolveToSignalObject=off  IntegratorRTWStateStorageClass=Auto  FilterContinuousStateAttributes=''  FilterStateMustResolveToSignalObject=off  FilterRTWStateStorageClass=Auto  DifferentiatorICPrevScaledInput=0  DifferentiatorOutMin=[]  DifferentiatorOutMax=[]
  PID Controller9 : simulink/Continuous/PID Controller  Controller=P  TimeDomain=Continuous-time  SampleTime=-1  IntegratorMethod=Forward Euler  FilterMethod=Forward Euler  Form=Parallel  UseFilter=on  ControllerParametersSource=internal  P=8  I=0  D=0  N=100  InitialConditionSource=internal  InitialConditionForIntegrator=0  InitialConditionForFilter=0  ExternalReset=none  LimitOutput=off  UpperSaturationLimit=inf  LowerSaturationLimit=-inf  LinearizeAsGain=on  AntiWindupMode=none  Kb=1  TrackingMode=off  Kt=1  PParamMin=[]  PParamMax=[]  IParamMin=[]  IParamMax=[]  DParamMin=[]  DParamMax=[]  NParamMin=[]  NParamMax=[]  KbParamMin=[]  KbParamMax=[]  KtParamMin=[]  KtParamMax=[]  POutMin=[]  POutMax=[]  IOutMin=[]  IOutMax=[]  DOutMin=[]  DOutMax=[]  NOutMin=[]  NOutMax=[]  KbOutMin=[]  KbOutMax=[]  KtOutMin=[]  KtOutMax=[]  IntegratorOutMin=[]  IntegratorOutMax=[]  FilterOutMin=[]  FilterOutMax=[]  SumOutMin=[]  SumOutMax=[]  SumI1OutMin=[]  SumI1OutMax=[]  SumI2OutMin=[]  SumI2OutMax=[]  SumI3OutMin=[]  SumI3OutMax=[]  SumDOutMin=[]  SumDOutMax=[]  SaturationOutMin=[]  SaturationOutMax=[]  IntegratorContinuousStateAttributes=''  IntegratorStateMustResolveToSignalObject=off  IntegratorRTWStateStorageClass=Auto  FilterContinuousStateAttributes=''  FilterStateMustResolveToSignalObject=off  FilterRTWStateStorageClass=Auto  DifferentiatorICPrevScaledInput=0  DifferentiatorOutMin=[]  DifferentiatorOutMax=[]
  Scope52 : Scope
  Scope58 : Scope
  Scope59 : Scope
  Sum : Sum  Inputs=|++
  Sum1 : Sum  Inputs=|++
  Sum3 : Sum  Inputs=|++
  e_Wx : Scope
  e_Wy : Scope
  e_Wz : Scope
  Out1 : Outport
  Out2 : Outport  Port=2
  Out3 : Outport  Port=3
  wires:
  PID Controller9/1 -> Scope52/1, Sum/2  "X"
  PID Controller11/1 -> Scope58/1, Sum3/2  "Z"
  PID Controller10/1 -> Sum1/2  "Y"
  Gain1/1 -> Derivative1/1
  In1/1 -> Demux4/1
  Demux4/3 -> Gain3/1, e_Wz/1, PID Controller11/1
  Demux4/2 -> e_Wy/1, Gain1/1, PID Controller10/1
  Derivative/1 -> Sum/1
  Gain/1 -> Derivative/1
  Derivative1/1 -> Sum1/1
  Sum1/1 -> Out2/1
  Demux4/1 -> e_Wx/1, Gain/1, PID Controller9/1
  Sum/1 -> Out1/1
  Gain3/1 -> Derivative3/1
  Derivative3/1 -> Sum3/1
  Sum3/1 -> Out3/1, Scope59/1

== system finishi/滤波器 KF/KF滤波/KF ==
  传感器位置 : Inport
  传感器加速度 : Inport  Port=2
  R矩阵 : Inport  Port=3
  KF : MATLAB Function  TreatAsAtomicUnit=on
  滤波后位置 : Outport
  滤波后速度 : Outport  Port=2
  wires:
  KF/1(P) -> 滤波后位置/1  "位置"
  传感器位置/1 -> KF/1(p)
  KF/2(V) -> 滤波后速度/1  "速度"
  传感器加速度/1 -> KF/2(a)
  R矩阵/1 -> KF/3(R)

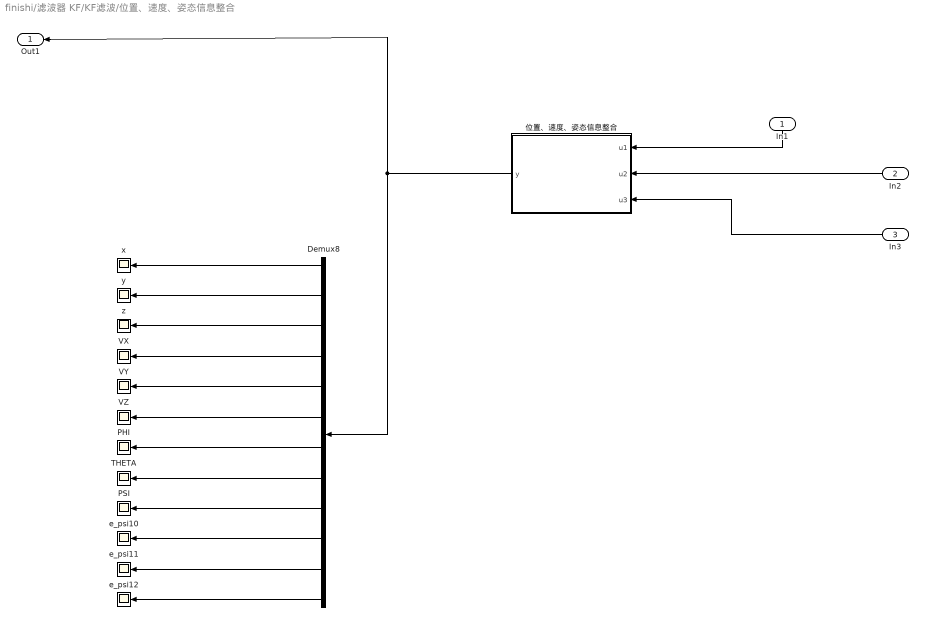
== system finishi/滤波器 KF/KF滤波/位置、速度、姿态信息整合 ==
  In1 : Inport
  In2 : Inport  Port=2
  In3 : Inport  Port=3
  Demux8 : Demux  Outputs=12
  PHI : Scope
  PSI : Scope
  THETA : Scope
  VX : Scope
  VY : Scope
  VZ : Scope
  e_psi10 : Scope
  e_psi11 : Scope
  e_psi12 : Scope
  x : Scope
  y : Scope
  z : Scope
  位置、速度、姿态信息整合 : MATLAB Function  TreatAsAtomicUnit=on
  Out1 : Outport
  wires:
  In2/1 -> 位置、速度、姿态信息整合/2(u2)
  In3/1 -> 位置、速度、姿态信息整合/3(u3)
  位置、速度、姿态信息整合/1(y) -> Out1/1, Demux8/1
  Demux8/1 -> x/1
  Demux8/4 -> VX/1
  Demux8/5 -> VY/1
  Demux8/6 -> VZ/1
  Demux8/2 -> y/1
  Demux8/7 -> PHI/1
  Demux8/3 -> z/1
  Demux8/12 -> e_psi12/1
  Demux8/11 -> e_psi11/1
  Demux8/9 -> PSI/1
  Demux8/8 -> THETA/1
  Demux8/10 -> e_psi10/1
  In1/1 -> 位置、速度、姿态信息整合/1(u1)

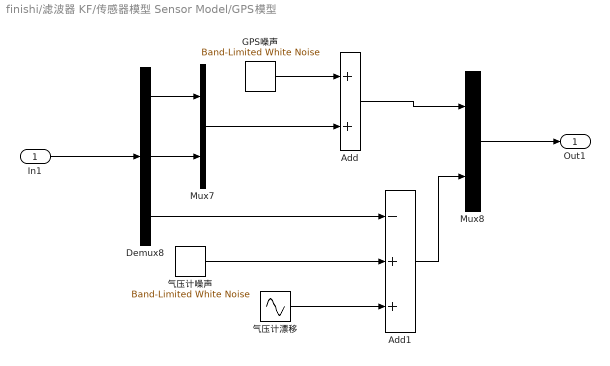
== system finishi/滤波器 KF/传感器模型 Sensor Model/GPS模型 ==
  In1 : Inport
  Add : Sum
  Add1 : Sum  Inputs=-++
  Demux8 : Demux  Outputs=3
  GPS噪声 : simulink/Sources/Band-Limited White Noise  Cov=[0.01;0.01]  Ts=0.01  seed=[23341]
  Mux7 : Mux  Inputs=2
  Mux8 : Mux  Inputs=2
  气压计噪声 : simulink/Sources/Band-Limited White Noise  Cov=[0.01]  Ts=0.01  seed=[23341]
  气压计漂移 : Sin  Amplitude=0.5  Frequency=0.05  SampleTime=0.01
  Out1 : Outport
  wires:
  气压计漂移/1 -> Add1/3
  Mux7/1 -> Add/2
  Demux8/3 -> Add1/1
  GPS噪声/1 -> Add/1
  In1/1 -> Demux8/1
  Add/1 -> Mux8/1
  Demux8/1 -> Mux7/1
  Demux8/2 -> Mux7/2
  Mux8/1 -> Out1/1
  Add1/1 -> Mux8/2
  气压计噪声/1 -> Add1/2

== system finishi/滤波器 KF/传感器模型 Sensor Model/加速度计模型 ==
  准确加速度 : Inport
  机体角度 : Inport  Port=2
  Add2 : Sum  Inputs=+--+
  MATLAB Function2 : MATLAB Function  TreatAsAtomicUnit=on
  g : Constant  Value=[0;0;9.8]
  加速度计噪声 : simulink/Sources/Band-Limited White Noise  Cov=[0.0001;0.0001;0.0001]  Ts=0.01  seed=[23341]
  加速度计漂移 : Subsystem
  欧拉角 : MATLAB Function  TreatAsAtomicUnit=on
  精确加速度 : MATLAB Function  TreatAsAtomicUnit=on
  传感器测量的加速度 : Outport
  wires:
  加速度计漂移/1(Out1) -> ?
  Add2/1 -> 传感器测量的加速度/1
  MATLAB Function2/1(y) -> Add2/4
  g/1 -> MATLAB Function2/1(u1)
  加速度计噪声/1 -> Add2/2
  准确加速度/1 -> 精确加速度/2(u2)
  欧拉角/1(y) -> MATLAB Function2/2(u2)
  机体角度/1 -> 欧拉角/1(u), 精确加速度/1(u1)
  精确加速度/1(y) -> Add2/1

== system finishi/滤波器 KF/传感器模型 Sensor Model/加速度计模型/加速度计漂移 ==
  Mux9 : Mux  Inputs=3
  气压计漂移1 : Sin  Amplitude=0.1  Frequency=0.05  SampleTime=0.01
  气压计漂移2 : Sin  Amplitude=0.1  Frequency=0.05  Phase=1  SampleTime=0.01
  气压计漂移3 : Sin  Amplitude=0.1  Frequency=0.05  Phase=2  SampleTime=0.01
  Out1 : Outport
  wires:
  Mux9/1 -> Out1/1
  气压计漂移1/1 -> Mux9/1
  气压计漂移3/1 -> Mux9/3
  气压计漂移2/1 -> Mux9/2

== matlab function finishi/八旋翼模型 Octorotor Model/控制刚体模型 Rigid Body Dynamcis ==
  data: u1 input; y output; u2 input; u3 input
function y = fcn(u1,u2,u3)
%#codegen
%%u1：转速的平方
%%u2：上一次计算后积分得到的数
%%u3：转速

%%初始化参数
m=5;
g=9.8;
Jxx=0.1539;
Jyy=0.1539;
Jzz=0.2634;
d=0.4;
CT=2.757*10^(-5);
CM=4.308*10^(-7);
CR=727.36;
Wb=173.03;
Jm=8.61*10^(-5);
Tm=0.0435;
Cd=0.712;

%%取输入参数
Ve=u2(4:6,1);
phi=u2(7);
theta=u2(8);
psi=u2(9);
Wb=u2(10:12,1);
JRP=Jm;
Wxb=u2(10,1);
Wyb=u2(11,1);
tau=u1(2:4,1);

Wk_1=u3(1);
Wk_2=u3(2);
Wk_3=u3(3);
Wk_4=u3(4);
Wk_5=u3(5);
Wk_6=u3(6);
Wk_7=u3(7);
Wk_8=u3(8);


%%速度
Pe_daoshu=Ve;

%%加速度
f=u1(1);%取输入中的力

R=[cos(theta)*cos(psi) cos(psi)*sin(theta)*sin(phi)-sin(psi)*cos(phi) cos(psi)*sin(theta)*cos(phi)+sin(psi)*sin(phi);...
   cos(theta)*sin(psi) sin(psi)*sin(theta)*sin(phi)+cos(psi)*cos(phi) sin(psi)*sin(theta)*cos(phi)-cos(psi)*sin(phi);...
   -sin(theta) sin(phi)*cos(theta) cos(phi)*cos(theta)];%%旋转矩阵
e3=[0 0 1]';%%取地面Z轴
Ve_daoshu=g.*e3-f/m.*R*e3;%%加速度

%%角速度
W=[1 0 -sin(theta);...
   0 cos(phi) cos(theta)*sin(phi);...
   0 -sin(phi) cos(theta)*cos(phi);]; %%欧拉角速度到机体角速度的转换
W_jiti=W*Wb;%%机体角速度

%%角加速度
J=[Jxx 0 0;...
   0 Jyy 0;...
   0 0 Jzz];%%转动惯量矩阵
Ga_phi=JRP*Wyb*Wk_1-JRP*Wyb*Wk_2+JRP*Wyb*Wk_3-JRP*Wyb*Wk_4+JRP*Wyb*Wk_5-JRP*Wyb*Wk_6+JRP*Wyb*Wk_7-JRP*Wyb*Wk_8;
Ga_theta=-(JRP*Wxb*Wk_1-JRP*Wxb*Wk_2+JRP*Wxb*Wk_3-JRP*Wxb*Wk_4+JRP*Wxb*Wk_5-JRP*Wxb*Wk_6+JRP*Wxb*Wk_7-JRP*Wxb*Wk_8);
Ga_psi=0;
Ga=[Ga_phi;Ga_theta;Ga_psi];
Wb_daoshu=J^(-1)*((cross((-Wb),(J*Wb)))+Ga+tau);

%%输出
y=[Pe_daoshu;Ve_daoshu;W_jiti;Wb_daoshu];

== matlab function finishi/八旋翼模型 Octorotor Model/控制效率模型 Power Model ==
  data: u input; y output
function y = fcn(u)
%#codegen
%%初始化
m=5;
g=9.8;
Jxx=0.1539;
Jyy=0.1539;
Jzz=0.2634;
d=0.4;
CT=2.757*10^(-5);
CM=4.308*10^(-7);
CR=727.36;
Wb=173.03;
Jm=8.61*10^(-5);
Tm=0.0435;
Cd=0.712;



w=u.^2;
apha1=pi/8;
apha2=apha1+pi/4;
apha3=apha2+pi/4;
apha4=apha3+pi/4;
apha5=apha4+pi/4;
apha6=apha5+pi/4;
apha7=apha6+pi/4;
apha8=apha7+pi/4;

Mnr=[CT CT CT CT CT CT CT CT;...
    -d*CT*sin(apha1) -d*CT*sin(apha2) -d*CT*sin(apha3) -d*CT*sin(apha4) -d*CT*sin(apha5) -d*CT*sin(apha6) -d*CT*sin(apha7) -d*CT*sin(apha8);...
    d*CT*cos(apha1) d*CT*cos(apha2) d*CT*cos(apha3) d*CT*cos(apha4) d*CT*cos(apha5) d*CT*cos(apha6) d*CT*cos(apha7) d*CT*cos(apha8);...
    CM -CM CM -CM CM -CM CM -CM];%%控制效率矩阵
FT=Mnr*w;%%力于力矩矩阵
y =FT;

== matlab function finishi/八旋翼模型 Octorotor Model/信号输出 Output/Px ==
  data: u input; y output
function y= fcn(u)
%#codegen
%%Vx
y = u(1);

== matlab function finishi/八旋翼模型 Octorotor Model/信号输出 Output/Py ==
  data: u input; y output
function y= fcn(u)
%#codegen
%%Vx
y = u(2);

== matlab function finishi/八旋翼模型 Octorotor Model/信号输出 Output/Pz ==
  data: u input; y output
function y= fcn(u)
%#codegen
%%Vx
y = u(3);

== matlab function finishi/八旋翼模型 Octorotor Model/信号输出 Output/Vx ==
  data: u input; y output
function y= fcn(u)
%#codegen
%%Vx
y = u(4);

== matlab function finishi/八旋翼模型 Octorotor Model/信号输出 Output/Vy ==
  data: u input; y output
function y= fcn(u)
%#codegen
%%Vx
y = u(5);

== matlab function finishi/八旋翼模型 Octorotor Model/信号输出 Output/Vz ==
  data: u input; y output
function y= fcn(u)
%#codegen
%%Vx
y = u(6);

== matlab function finishi/八旋翼模型 Octorotor Model/信号输出 Output/phi ==
  data: u input; y output
function y= fcn(u)
%#codegen
%%Vx
y = u(7);

== matlab function finishi/八旋翼模型 Octorotor Model/信号输出 Output/theta ==
  data: u input; y output
function y= fcn(u)
%#codegen
%%Vx
y = u(8);

== matlab function finishi/八旋翼模型 Octorotor Model/信号输出 Output/psi ==
  data: u input; y output
function y= fcn(u)
%#codegen
%%Vx
y = u(9);

== matlab function finishi/八旋翼模型 Octorotor Model/信号输出 Output/phi' ==
  data: u input; y output
function y= fcn(u)
%#codegen
%%Vx
y = u(10);

== matlab function finishi/八旋翼模型 Octorotor Model/信号输出 Output/theta' ==
  data: u input; y output
function y= fcn(u)
%#codegen
%%Vx
y = u(11);

== matlab function finishi/八旋翼模型 Octorotor Model/信号输出 Output/psi' ==
  data: u input; y output
function y= fcn(u)
%#codegen
%%Vx
y = u(12);

== matlab function finishi/底层控制器 Low-Level Controller/位置控制器 Position Controller/fd1 ==
  data: u input; y output
function y= fcn(u)
%#codegen
%%fd
y = u(3);

== matlab function finishi/底层控制器 Low-Level Controller/位置控制器 Position Controller/位置误差解算1 ==
  data: u1 input; y output; u2 input
function y = fcn(u1,u2)
%#codegen
%%u1为目标位置
%%u2为当前位置、姿态信息

%%设置初始参数
Kph_x=1.55;      %x方向的P调节
a1_x=10;       %x方向的误差饱和限制
Kph_y=1.55;      %y方向的P调节
a1_y=10;       %y方向的误差饱和限制
Kpz=4;        %z方向的P调节
a4=10;         %z方向的误差饱和限制


%%取目标参数
Phd_x=u1(1);   %x方向的目标位置值
Phd_y=u1(2);   %y方向的目标位置值
Pzd=u1(3);     %z方向的目标位置值


%取当前参数
Ph_x=u2(1);    %x方向的当前位置值
Vh_x=u2(4);    %x方向的当前速度值
Ph_y=u2(2);    %y方向的当前位置值
Vh_y=u2(5);    %y方向的当前速度值
Pz=u2(3);      %z方向的当前位置值
Vz=u2(6);      %z方向的当前速度值


%%水平位置通道
Vhd_x=Kph_x*(Phd_x-Ph_x);
evh_x=sat((Vh_x-Vhd_x),a1_x);

Vhd_y=Kph_y*(Phd_y-Ph_y);
evh_y=sat((Vh_y-Vhd_y),a1_y);

%%高度通道
Vzd=-Kpz*(Pz-Pzd);
evz=sat((Vz-Vzd),a4);


y=[evh_x evh_y evz]';

== matlab function finishi/底层控制器 Low-Level Controller/姿态控制器 Attitude Controller/姿态误差解算1 ==
  data: u1 input; y output; u2 input; u3 input
function y = fcn(u1,u2,u3)
%#codegen
%%u1为目标姿态角
%%u2为给定的偏航角
%%u3为当前位置、姿态信息

%%设置初始参数
  %%phi的参数设置
K_phi=8;     %P调节
a10_x=20;     %误差饱和限制

  %%theta的参数设置
K_theta=8;     %P调节
a10_y=20;     %误差饱和限制

  %%psi的参数设置
K_psi=2.6;     %P调节
a10_z=10;     %误差饱和限制
          
%g=9.8;
%m=5;


%%取当前的姿态参数
phi=u3(7);
psi=u3(9);
theta=u3(8);

W_x=u3(10);
W_y=u3(11);
W_z=u3(12);

%%取目标姿态角
phi_d=u1(1);
theta_d=u1(2);
psi_d=u2;

%%phi角度通道
e_phi=phi-phi_d;
Wd_x=-K_phi*e_phi;
eW_x=sat((W_x-Wd_x),a10_x);

%%theta角度通道
e_theta=theta-theta_d;
Wd_y=-K_theta*e_theta;
eW_y=sat((W_y-Wd_y),a10_y);

%%psi角度通道
e_psi=psi-psi_d;
%e_psi=sat(e_psi,pi/6);
Wd_z=-K_psi*e_psi;
eW_z=sat((W_z-Wd_z),a10_z);


y=[eW_x eW_y eW_z]';

== matlab function finishi/底层控制器 Low-Level Controller/位置控制器 Position Controller/输出目标theta phi角度1 ==
  data: u1 input; y output; u2 input; u3 input; u4 input
function y = fcn(u1,u2,u3,u4)
%#codegen
%%u1为X
%%u2为Y
%%u3为Z
%%u4为当前位置、姿态信息

%%设置初始参数
a2_phi=pi/4;       %phi角度的误差饱和限制
a2_theta=pi/4;       %theta角度的误差饱和限制
a5=200;            %推力的饱和限制
g=9.8;
m=5;


%%取参数
X=u1;
Y=u2;
Z=u3;
psi=u4(9);


%%水平位置通道
phi=sat(((1)*g^(-1)*(sin(psi)*X-cos(psi)*Y)),a2_phi);
theta=sat(((1)*g^(-1)*(cos(psi)*X+sin(psi)*Y)),a2_theta);
fd=sat((m*(g+Z)),a5);

y=[phi theta fd]';

== matlab function finishi/底层控制器 Low-Level Controller/姿态控制器 Attitude Controller/输出目标力矩1 ==
  data: u1 input; y output; u2 input; u3 input
function y = fcn(u1,u2,u3)
%#codegen
%%u1为tau_x
%%u2为tau_y
%%u3为tao_z


%%设置初始参数
a11_x=60;       %x力矩的饱和限制
a11_y=60;       %y力矩的饱和限制
a11_z=10;       %z力矩的饱和限制


%%取参数
tau_x=-u1;
tau_y=-u2;
tau_z=-u3;



%%水平位置通道
tau_dx=sat((tau_x),a11_x);
tau_dy=sat((tau_y),a11_y);
tau_dz=sat((tau_z),a11_z);
y=[tau_dx tau_dy tau_dz]';

== matlab function finishi/八旋翼模型 Octorotor Model/信号输出 Output/总速度  ==
  data: u1 input; y output; u2 input; u3 input
function y = fcn(u1,u2,u3)
%#codegen
%%u1：Vx
%%u2：Vy
%%u3：Vz

%%初始化参数

%%取输入参数
Vx=u1;
Vy=u2;
Vz=u3;
%%速度
V=(Vx^2+Vy^2+Vz^2)^(0.5);


%%输出
y=V;

== matlab function finishi/决策模块 Decision/决策 Decision ==
  data: u1 input; y output; u2 input
function y = fcn(u1, u2)

%#codegen
%取参数
P=u1(1:3,1);%当前位置
t=u2;
%计算
persistent k;
if isempty(k)
    k=1;
end

persistent j;
if isempty(j)
    j=0;
end

persistent i;
if isempty(i)
    i=0;
end

persistent P_home;
if isempty(P_home)
    P_home=[0;0;0];
end

P_wp=[0 0 10 10 20 20 30 30 40 40;...
      0 100 100 0 0 100 100 0 0 100; 
      -1 -1 -1 -1 -1 -1 -1 -1 -1 -1];
  
  persistent P_wp_cur;
if isempty(P_wp_cur)
    P_wp_cur=[0;0;-1];
end
  
persistent t_home;
if isempty(t_home)
    t_home=0;
end

  ipsilong=0.01;

  if t~=0 && mod((t-t_home),100)==0%%%%%%%%%%%%%%%%%%%没电
      t_meidianhuijia=t
      i=1;
      j=1;
      P_home=P;
      P_wp_cur=[0;0;-1];  
  else%%%%%%%%%%%%%%%%%%%%%%有电
      if norm(P_wp_cur-P)>ipsilong%%%%%%%%%%%%%%%%%%%%%%%没进入航点
      else%%%%%%%%%%%%%%%%%%%进入航点
          if i==1%%%%%%%%%%%%%%回家中
              if j==0%%回家结束
                  i=0;
                  P_wp_cur=P_wp(1:3,k);
                  t_chongdianhuiyuanlu=t
                   
              else %%回家半路
                  P_wp_cur=P_home;
                  j=0;
                  t_home=t;
                  t_chongdian=t
                  t;
              end
          else%%%%%%%%%%%%%不在回家中
              if k==10%%%%%完成了
                  P_wp_cur=[0;0;-1];
                  t_wanchengrenwu=t

                  k=k+1;

              else%%%未完成
                  k=k+1;
                  P_wp_cur=P_wp(1:3,k);
                 
              end
          end
      end
  end
  
if norm(P_wp_cur-P)>=1
    P_wp_cur_xiao=(P_wp_cur-P).*(1/(norm(P_wp_cur-P)))+P;
else
    P_wp_cur_xiao=P_wp_cur;
end
  y=P_wp_cur_xiao;
end

== matlab function finishi/底层控制器 Low-Level Controller/控制分配器 Control Allocator /控制分配：输出转速 ==
  data: u1 input; y output; u2 input
function y = fcn(u1,u2)
%#codegen
%%u1为fd
%%u2为力矩

%%初始化
m=5;
g=9.8;
Jxx=0.1539;
Jyy=0.1539;
Jzz=0.2634;
d=0.4;
CT=2.757*10^(-5);
CM=4.308*10^(-7);
CR=727.36;
Wb=173.03;
Jm=8.61*10^(-5);
Tm=0.0435;
Cd=0.712;

apha1=pi/8;
apha2=apha1+pi/4;
apha3=apha2+pi/4;
apha4=apha3+pi/4;
apha5=apha4+pi/4;
apha6=apha5+pi/4;
apha7=apha6+pi/4;
apha8=apha7+pi/4;

M8=[CT CT CT CT CT CT CT CT;...
    -d*CT*sin(apha1) -d*CT*sin(apha2) -d*CT*sin(apha3) -d*CT*sin(apha4) -d*CT*sin(apha5) -d*CT*sin(apha6) -d*CT*sin(apha7) -d*CT*sin(apha8);...
    d*CT*cos(apha1) d*CT*cos(apha2) d*CT*cos(apha3) d*CT*cos(apha4) d*CT*cos(apha5) d*CT*cos(apha6) d*CT*cos(apha7) d*CT*cos(apha8);...
    CM -CM CM -CM CM -CM CM -CM];%%控制效率矩阵

%%解算
P8=M8'*((M8*(M8'))^(-1));%%伪逆矩阵
ftau=[u1;u2(1);u2(2);u2(3)];
w2=P8*ftau;

w=zeros(8,1);

for i=1:8
    if w2(i)>=0
        w(i)=w2(i).^(0.5);
    else
        w(i)=0;
    end
end
        
y=w;

== matlab function finishi/底层控制器 Low-Level Controller/电机控制：输出油门 Rotor Controller ==
  data: u1 input; y output
function y = fcn(u1)
%#codegen
%%u1为转速


%%初始化
m=5;
g=9.8;
Jxx=0.1539;
Jyy=0.1539;
Jzz=0.2634;
d=0.4;
CT=2.757*10^(-5);
CM=4.308*10^(-7);
CR=727.36;
Wb=173.03;
Jm=8.61*10^(-5);
Tm=0.0435;
Cd=0.712;

%%取输入
Wss=u1;


%%解算
youmen=(Wss-Wb.*ones(8,1)).*(1/CR);
youmen_baohe=zeros(8,1);
for i=1:8
    if youmen(i)>=0&&youmen(i)<=1
        youmen_baohe(i,1)=youmen(i);
    else if youmen(i)>1
           youmen_baohe(i,1)=1;
        else 
            youmen_baohe(i,1)=0;
        end
    end
end


y=youmen_baohe;

== matlab function finishi/八旋翼模型 Octorotor Model/信号输出 Output/ax1 ==
  data: u input; y output
function y= fcn(u)
%#codegen
%%Vx
y = u(4);

== matlab function finishi/八旋翼模型 Octorotor Model/信号输出 Output/ay1 ==
  data: u input; y output
function y= fcn(u)
%#codegen
%%Vx
y = u(5);

== matlab function finishi/八旋翼模型 Octorotor Model/信号输出 Output/az1 ==
  data: u input; y output
function y= fcn(u)
%#codegen
%%Vx
y = u(6);

== matlab function finishi/八旋翼模型 Octorotor Model/信号输出 Output/R矩阵 ==
  data: u1 input; y output; u2 input; u3 input
function y = fcn(u1,u2,u3)
%#codegen
%%u1：phi
%%u2：theta
%%u3：psi

%%取参数
phi=u1;
theta=u2;
psi=u3;

R=[cos(theta)*cos(psi) cos(psi)*sin(theta)*sin(phi)-sin(psi)*cos(phi) cos(psi)*sin(theta)*cos(phi)+sin(psi)*sin(phi);...
   cos(theta)*sin(psi) sin(psi)*sin(theta)*sin(phi)+cos(psi)*cos(phi) sin(psi)*sin(theta)*cos(phi)-cos(psi)*sin(phi);...
   -sin(theta) sin(phi)*cos(theta) cos(phi)*cos(theta)];%%旋转矩阵

%%输出
y=R;

== matlab function finishi/滤波器 KF/KF滤波/位置、速度、姿态信息整合/位置、速度、姿态信息整合 ==
  data: u1 input; y output; u2 input; u3 input
function y = fcn(u1,u2,u3)
%#codegen
%%u1为姿态
%%u2为位置
%%u3为速度
canshu=u1;
y = u1;

== matlab function finishi/滤波器 KF/KF滤波/KF/KF ==
  data: p input; P output; a input; R input; V output
function [P,V] = fcn(p,a,R)

p=p.*[1;1;-1];
a=R*a-[0;0;9.8];
persistent Xt;
persistent Vt;
persistent Mt;
persistent a_last;
if isempty(a_last)
    a_last=zeros(3,1);
end
I=eye(3);
O=zeros(3);
dt=0.01;
if isempty(Xt)
    Xt=zeros(3,1);
end
if isempty(Vt)
    Vt=zeros(3,1);
end
if isempty(Mt)
    Mt=[2*I,   O;
        O,     I];
end
Gt=[I,dt*I;
   O,   I ];
Ht=[I,    O; 
    I./dt,O];
Ra=[0.01,0,0;
    0,0.01,0;
    0,0,0.01];
Rv=dt*R*Ra;
Rx=dt*Rv;
Rt=[Rx,O;
    O,Rv];
Qp=[1,0,0;
    0,1,0;
    0,0,1];
Qt=[Qp,  O;
    O,   O];
X_t=Xt+Vt.*dt;
V_t=Vt+a_last.*dt;
M_t=Gt*Mt*Gt'+Rt;
Kt=M_t*Ht'*inv(Ht*M_t*Ht'+Qt);
Zp=p;
Zv=zeros(3,1);
Zt=[Zp;Zv];
hp=X_t;
hv=zeros(3,1);
ht=[hp;hv];
Ut=[X_t;V_t]+Kt*(Zt-ht);
Mt=(eye(6)-Kt*Ht)*M_t;
Xt=[Ut(1,1);Ut(2,1);Ut(3,1)];
Vt=[Ut(4,1);Ut(5,1);Ut(6,1)];
a_last=a;
P=Xt;
V=Vt;
end

== matlab function finishi/滤波器 KF/传感器模型 Sensor Model/加速度计模型/MATLAB Function2 ==
  data: u1 input; y output; u2 input
function y = fcn(u1,u2)
%#codegen
%%计算g在体轴系中的影响

%%u1为加速度
%%u2为欧拉角

%%取参数
g=u1;
phi=u2(1);
theta=u2(2);
psi=u2(3);

%%计算
R=[cos(theta)*cos(psi) cos(psi)*sin(theta)*sin(phi)-sin(psi)*cos(phi) cos(psi)*sin(theta)*cos(phi)+sin(psi)*sin(phi);...
   cos(theta)*sin(psi) sin(psi)*sin(theta)*sin(phi)+cos(psi)*cos(phi) sin(psi)*sin(theta)*cos(phi)-cos(psi)*sin(phi);...
   -sin(theta) sin(phi)*cos(theta) cos(phi)*cos(theta)];%%旋转矩阵

g_b=R^(-1)*g;
y = g_b;

== matlab function finishi/滤波器 KF/传感器模型 Sensor Model/加速度计模型/欧拉角 ==
  data: u input; y output
function y = fcn(u)
%#codegen
%%计算欧拉角

%%u为机体角度

%%取参数
phi=u(1);
theta=u(2);
psi=u(3);
w_b=u;

%%计算
W=[1   tan(theta)*sin(phi)    tan(theta)*cos(phi);
   0   cos(phi)              -sin(phi);
   0   sin(phi)/cos(theta)    cos(phi)/cos(theta);];
Euler=W*w_b;


y = Euler;

== matlab function finishi/滤波器 KF/传感器模型 Sensor Model/加速度计模型/精确加速度 ==
  data: u1 input; y output; u2 input
function y = fcn(u1,u2)
%#codegen

%%u1为机体角度
%%u2为地轴系加速度

%%取参数
phi=u1(1);
theta=u1(2);
psi=u1(3);
a_e=u2;

%%计算
R=[cos(theta)*cos(psi) cos(psi)*sin(theta)*sin(phi)-sin(psi)*cos(phi) cos(psi)*sin(theta)*cos(phi)+sin(psi)*sin(phi);...
   cos(theta)*sin(psi) sin(psi)*sin(theta)*sin(phi)+cos(psi)*cos(phi) sin(psi)*sin(theta)*cos(phi)-cos(psi)*sin(phi);...
   -sin(theta) sin(phi)*cos(theta) cos(phi)*cos(theta)];%%旋转矩阵
a_b=R^(-1)*a_e;


y = a_b;
